simulink model "fourWheelRobotControl_v1"  (R2020b)
settings: Solver=ode3  StartTime=0.0  StopTime=tf  FixedStep=0.0001  RelTol=1e-4  EnableMultiTasking=on
values from neighbouring files (symbols this model uses):
  k_E = 1    [main_robot_control_simulation.m]
  p = [0.127,0.7,0.7,25,0.68,0.001,0.99,0.015,Kt,0.002*Kt,0.56*Kt,     0.00024*Kt,100,0.01,19.2,0,pi/4,-pi/4,pi/4,-pi/4,0,0,0,0]    [main_robot_control_simulation.m]
libraries: pid_lib x7
settings Model: Creator=Sarot PC  LastModifiedBy=ONLY-GOD
settings DataIOCC: LimitDataPoints=on  SaveFormat=Array  ReturnWorkspaceOutputs=off
settings OptimizationCC: LifeSpan=inf
settings DebuggingCC: SolverPrmCheckMsg=warning  InheritedTsInSrcMsg=none  TasksWithSamePriorityMsg=none  SigSpecEnsureSampleTimeMsg=none  ParameterOverflowMsg=none  SignalLabelMismatchMsg=warning  SFUnexpectedBacktrackingDiag=warning  SFNoUnconditionalDefaultTransitionDiag=warning  SFExecutionAtInitializationDiag=none  ArithmeticOperatorsInVariantConditions=warning
settings HardwareCC: ProdBitPerPointer=32  ProdBitPerSizeT=32  ProdBitPerPtrDiffT=32  ProdLargestAtomicFloat=None  ProdIntDivRoundTo=Undefined  ProdEndianess=Unspecified  ProdWordSize=32  ProdHWDeviceType=32-bit Generic
settings ModelReferenceCC: PropagateSignalLabelsOutOfModel=off
settings SFSimCC: SimUseLocalCustomCode=off  CustomCodeUndefinedFunction=UseInterfaceOnly
settings RTWCC: RTWUseLocalCustomCode=off
settings CodeAppCC: StateflowObjectComments=on
settings GRTTargetCC: TargetLangStandard=C89/C90 (ANSI)
settings ConfigComp: CovMetricSettings=dw  CovSaveCumulativeToWorkspaceVar=on  CovSaveSingleToWorkspaceVar=on  CovExternalEMLEnable=off  CovSFcnEnable=off

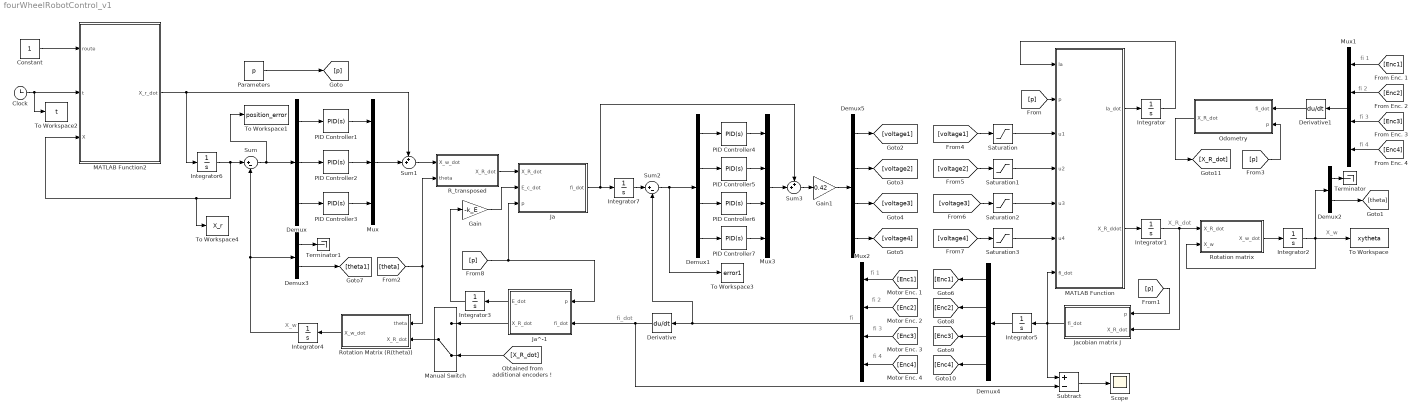
== system fourWheelRobotControl_v1 ==
  note: fi 4
  note: fi 3
  note: fi 2
  note: fi 1
  note: fi_dot
  note: fi
  note: X_w
  note: X_w
  note: X_R_dot
  note: fi 4
  note: fi 3
  note: fi 2
  note: fi 1
  Clock : Clock
  Constant : Constant
  Demux : Demux  Outputs=3
  Demux1 : Demux
  Demux2 : Demux  Outputs=[2,1]
  Demux3 : Demux  Outputs=[2,1]
  Demux4 : Demux
  Demux5 : Demux
  Derivative : Derivative  CoefficientInTFapproximation=0.01
  Derivative1 : Derivative  CoefficientInTFapproximation=0.01
  Gain : Gain  Gain=-k_E
  Gain1 : Gain  Gain=0.42
  Integrator : Integrator  InitialCondition=[0;0;0;0]
  Integrator{1..2,4,6} (4 alike) : Integrator  InitialCondition=[0;0;0]
  Integrator3 : Integrator
  Integrator5 : Integrator  InitialCondition=[0;0;0;0]
  Integrator7 : Integrator  InitialCondition=[0;0;0;0]
  Ja : MATLAB Function  TreatAsAtomicUnit=on
  Ja^-1 : MATLAB Function  TreatAsAtomicUnit=on
  Jacobian matrix J : MATLAB Function  TreatAsAtomicUnit=on
  MATLAB Function : MATLAB Function  TreatAsAtomicUnit=on
  MATLAB Function2 : MATLAB Function  TreatAsAtomicUnit=on
  Manual Switch : ManualSwitch  CurrentSetting=0
  Mux : Mux  Inputs=3
  Mux1 : Mux
  Mux2 : Mux
  Mux3 : Mux
  Odometry : MATLAB Function  TreatAsAtomicUnit=on
  PID Controller1 : pid_lib/PID Controller  Controller=PID  Form=Parallel  TimeDomain=Continuous-time  UseExternalTs=off  SampleTime=-1  IntegratorMethod=Forward Euler  FilterMethod=Forward Euler  ControllerParametersSource=internal  P=5  I=5  D=0  UseFilter=on  N=1000  TunerSelectOption=Transfer Function Based (PID Tuner App)  InitialConditionSource=internal  InitialConditionForIntegrator=0  InitialConditionForFilter=0  DifferentiatorICPrevScaledInput=0  ExternalReset=none  TrackingMode=off  Kt=1  LimitOutput=off  SatLimitsSource=internal  UpperSaturationLimit=inf  LowerSaturationLimit=-inf  LinearizeAsGain=on  AntiWindupMode=none  Kb=1  POutMin=[]  POutMax=[]  IOutMin=[]  IOutMax=[]  DOutMin=[]  DOutMax=[]  NOutMin=[]  NOutMax=[]  SumOutMin=[]  SumOutMax=[]  SaturationOutMin=[]  SaturationOutMax=[]  PParamMin=[]  PParamMax=[]  IParamMin=[]  IParamMax=[]  DParamMin=[]  DParamMax=[]  NParamMin=[]  NParamMax=[]  KbParamMin=[]  KbParamMax=[]  KtParamMin=[]  KtParamMax=[]  KbOutMin=[]  KbOutMax=[]  KtOutMin=[]  KtOutMax=[]  IntegratorOutMin=[]  IntegratorOutMax=[]  FilterOutMin=[]  FilterOutMax=[]  SumI1OutMin=[]  SumI1OutMax=[]  SumI2OutMin=[]  SumI2OutMax=[]  SumI3OutMin=[]  SumI3OutMax=[]  SumI4OutMin=[]  SumI4OutMax=[]  SumDOutMin=[]  SumDOutMax=[]  DifferentiatorOutMin=[]  DifferentiatorOutMax=[]  FilterDiffOutCoefMin=[]  FilterDiffOutCoefMax=[]  ReciprocalOutMin=[]  ReciprocalOutMax=[]  SumDenOutMin=[]  SumDenOutMax=[]  SumNumOutMin=[]  SumNumOutMax=[]  DivideOutMin=[]  DivideOutMax=[]  UdiffTsProdOutMin=[]  UdiffTsProdOutMax=[]  NTsProdOutMin=[]  NTsProdOutMax=[]  UintegralTsProdOutMin=[]  UintegralTsProdOutMax=[]  UngainTsProdOutMin=[]  UngainTsProdOutMax=[]  IntegratorContinuousStateAttributes=''  IntegratorStateMustResolveToSignalObject=off  IntegratorRTWStateStorageClass=Auto  FilterContinuousStateAttributes=''  FilterStateMustResolveToSignalObject=off  FilterRTWStateStorageClass=Auto  ParallelPVariant=InternalParameters  IdealPVariant=Disabled  IVariant=InternalParameters  DVariant=InternalParameters  IntegratorVariant=Continuous  SatVariant=Disabled  AWVariant=Passthrough  PCopyVariant=Disabled  TRVariant=Disabled  FdbkBlocksVariant=Forward  IdealPFdbkVariant=Disabled  SatFdbkVariant=Disabled  DerivativeFilterVariant=ContFilter  NVariant=InternalParameters  NCopyVariant=Disabled  FilterICVariant=InternalICsFilter  IntegratorICVariant=InternalICs  ExternalResetVariant=Disabled  TRSumVariant=Passthrough  SumFdbkVariant=Disabled  SumVariant=Sum_PID  TsampFilterVariant=InternalTs  TsampNgainVariant=Passthrough  TsampIntegralVariant=Passthrough  ExternalSaturationOutDataTypeStr=Inherit: Same as second input
  PID Controller2 : pid_lib/PID Controller  Controller=PID  Form=Parallel  TimeDomain=Continuous-time  UseExternalTs=off  SampleTime=-1  IntegratorMethod=Forward Euler  FilterMethod=Forward Euler  ControllerParametersSource=internal  P=5  I=5  D=0  UseFilter=on  N=1000  TunerSelectOption=Transfer Function Based (PID Tuner App)  InitialConditionSource=internal  InitialConditionForIntegrator=0  InitialConditionForFilter=0  DifferentiatorICPrevScaledInput=0  ExternalReset=none  TrackingMode=off  Kt=1  LimitOutput=off  SatLimitsSource=internal  UpperSaturationLimit=inf  LowerSaturationLimit=-inf  LinearizeAsGain=on  AntiWindupMode=none  Kb=1  POutMin=[]  POutMax=[]  IOutMin=[]  IOutMax=[]  DOutMin=[]  DOutMax=[]  NOutMin=[]  NOutMax=[]  SumOutMin=[]  SumOutMax=[]  SaturationOutMin=[]  SaturationOutMax=[]  PParamMin=[]  PParamMax=[]  IParamMin=[]  IParamMax=[]  DParamMin=[]  DParamMax=[]  NParamMin=[]  NParamMax=[]  KbParamMin=[]  KbParamMax=[]  KtParamMin=[]  KtParamMax=[]  KbOutMin=[]  KbOutMax=[]  KtOutMin=[]  KtOutMax=[]  IntegratorOutMin=[]  IntegratorOutMax=[]  FilterOutMin=[]  FilterOutMax=[]  SumI1OutMin=[]  SumI1OutMax=[]  SumI2OutMin=[]  SumI2OutMax=[]  SumI3OutMin=[]  SumI3OutMax=[]  SumI4OutMin=[]  SumI4OutMax=[]  SumDOutMin=[]  SumDOutMax=[]  DifferentiatorOutMin=[]  DifferentiatorOutMax=[]  FilterDiffOutCoefMin=[]  FilterDiffOutCoefMax=[]  ReciprocalOutMin=[]  ReciprocalOutMax=[]  SumDenOutMin=[]  SumDenOutMax=[]  SumNumOutMin=[]  SumNumOutMax=[]  DivideOutMin=[]  DivideOutMax=[]  UdiffTsProdOutMin=[]  UdiffTsProdOutMax=[]  NTsProdOutMin=[]  NTsProdOutMax=[]  UintegralTsProdOutMin=[]  UintegralTsProdOutMax=[]  UngainTsProdOutMin=[]  UngainTsProdOutMax=[]  IntegratorContinuousStateAttributes=''  IntegratorStateMustResolveToSignalObject=off  IntegratorRTWStateStorageClass=Auto  FilterContinuousStateAttributes=''  FilterStateMustResolveToSignalObject=off  FilterRTWStateStorageClass=Auto  ParallelPVariant=InternalParameters  IdealPVariant=Disabled  IVariant=InternalParameters  DVariant=InternalParameters  IntegratorVariant=Continuous  SatVariant=Disabled  AWVariant=Passthrough  PCopyVariant=Disabled  TRVariant=Disabled  FdbkBlocksVariant=Forward  IdealPFdbkVariant=Disabled  SatFdbkVariant=Disabled  DerivativeFilterVariant=ContFilter  NVariant=InternalParameters  NCopyVariant=Disabled  FilterICVariant=InternalICsFilter  IntegratorICVariant=InternalICs  ExternalResetVariant=Disabled  TRSumVariant=Passthrough  SumFdbkVariant=Disabled  SumVariant=Sum_PID  TsampFilterVariant=InternalTs  TsampNgainVariant=Passthrough  TsampIntegralVariant=Passthrough  ExternalSaturationOutDataTypeStr=Inherit: Same as second input
  PID Controller3 : pid_lib/PID Controller  Controller=PID  Form=Parallel  TimeDomain=Continuous-time  UseExternalTs=off  SampleTime=-1  IntegratorMethod=Forward Euler  FilterMethod=Forward Euler  ControllerParametersSource=internal  P=5  I=5  D=0  UseFilter=on  N=1000  TunerSelectOption=Transfer Function Based (PID Tuner App)  InitialConditionSource=internal  InitialConditionForIntegrator=0  InitialConditionForFilter=0  DifferentiatorICPrevScaledInput=0  ExternalReset=none  TrackingMode=off  Kt=1  LimitOutput=off  SatLimitsSource=internal  UpperSaturationLimit=inf  LowerSaturationLimit=-inf  LinearizeAsGain=on  AntiWindupMode=none  Kb=1  POutMin=[]  POutMax=[]  IOutMin=[]  IOutMax=[]  DOutMin=[]  DOutMax=[]  NOutMin=[]  NOutMax=[]  SumOutMin=[]  SumOutMax=[]  SaturationOutMin=[]  SaturationOutMax=[]  PParamMin=[]  PParamMax=[]  IParamMin=[]  IParamMax=[]  DParamMin=[]  DParamMax=[]  NParamMin=[]  NParamMax=[]  KbParamMin=[]  KbParamMax=[]  KtParamMin=[]  KtParamMax=[]  KbOutMin=[]  KbOutMax=[]  KtOutMin=[]  KtOutMax=[]  IntegratorOutMin=[]  IntegratorOutMax=[]  FilterOutMin=[]  FilterOutMax=[]  SumI1OutMin=[]  SumI1OutMax=[]  SumI2OutMin=[]  SumI2OutMax=[]  SumI3OutMin=[]  SumI3OutMax=[]  SumI4OutMin=[]  SumI4OutMax=[]  SumDOutMin=[]  SumDOutMax=[]  DifferentiatorOutMin=[]  DifferentiatorOutMax=[]  FilterDiffOutCoefMin=[]  FilterDiffOutCoefMax=[]  ReciprocalOutMin=[]  ReciprocalOutMax=[]  SumDenOutMin=[]  SumDenOutMax=[]  SumNumOutMin=[]  SumNumOutMax=[]  DivideOutMin=[]  DivideOutMax=[]  UdiffTsProdOutMin=[]  UdiffTsProdOutMax=[]  NTsProdOutMin=[]  NTsProdOutMax=[]  UintegralTsProdOutMin=[]  UintegralTsProdOutMax=[]  UngainTsProdOutMin=[]  UngainTsProdOutMax=[]  IntegratorContinuousStateAttributes=''  IntegratorStateMustResolveToSignalObject=off  IntegratorRTWStateStorageClass=Auto  FilterContinuousStateAttributes=''  FilterStateMustResolveToSignalObject=off  FilterRTWStateStorageClass=Auto  ParallelPVariant=InternalParameters  IdealPVariant=Disabled  IVariant=InternalParameters  DVariant=InternalParameters  IntegratorVariant=Continuous  SatVariant=Disabled  AWVariant=Passthrough  PCopyVariant=Disabled  TRVariant=Disabled  FdbkBlocksVariant=Forward  IdealPFdbkVariant=Disabled  SatFdbkVariant=Disabled  DerivativeFilterVariant=ContFilter  NVariant=InternalParameters  NCopyVariant=Disabled  FilterICVariant=InternalICsFilter  IntegratorICVariant=InternalICs  ExternalResetVariant=Disabled  TRSumVariant=Passthrough  SumFdbkVariant=Disabled  SumVariant=Sum_PID  TsampFilterVariant=InternalTs  TsampNgainVariant=Passthrough  TsampIntegralVariant=Passthrough  ExternalSaturationOutDataTypeStr=Inherit: Same as second input
  PID Controller{4..7} (4 alike) : pid_lib/PID Controller  Controller=PID  Form=Parallel  TimeDomain=Continuous-time  UseExternalTs=off  SampleTime=-1  IntegratorMethod=Forward Euler  FilterMethod=Forward Euler  ControllerParametersSource=internal  P=100  I=0  D=30  UseFilter=on  N=1000  TunerSelectOption=Transfer Function Based (PID Tuner App)  InitialConditionSource=internal  InitialConditionForIntegrator=0  InitialConditionForFilter=0  DifferentiatorICPrevScaledInput=0  ExternalReset=none  TrackingMode=off  Kt=1  LimitOutput=off  SatLimitsSource=internal  UpperSaturationLimit=inf  LowerSaturationLimit=-inf  LinearizeAsGain=on  AntiWindupMode=none  Kb=1  POutMin=[]  POutMax=[]  IOutMin=[]  IOutMax=[]  DOutMin=[]  DOutMax=[]  NOutMin=[]  NOutMax=[]  SumOutMin=[]  SumOutMax=[]  SaturationOutMin=[]  SaturationOutMax=[]  PParamMin=[]  PParamMax=[]  IParamMin=[]  IParamMax=[]  DParamMin=[]  DParamMax=[]  NParamMin=[]  NParamMax=[]  KbParamMin=[]  KbParamMax=[]  KtParamMin=[]  KtParamMax=[]  KbOutMin=[]  KbOutMax=[]  KtOutMin=[]  KtOutMax=[]  IntegratorOutMin=[]  IntegratorOutMax=[]  FilterOutMin=[]  FilterOutMax=[]  SumI1OutMin=[]  SumI1OutMax=[]  SumI2OutMin=[]  SumI2OutMax=[]  SumI3OutMin=[]  SumI3OutMax=[]  SumI4OutMin=[]  SumI4OutMax=[]  SumDOutMin=[]  SumDOutMax=[]  DifferentiatorOutMin=[]  DifferentiatorOutMax=[]  FilterDiffOutCoefMin=[]  FilterDiffOutCoefMax=[]  ReciprocalOutMin=[]  ReciprocalOutMax=[]  SumDenOutMin=[]  SumDenOutMax=[]  SumNumOutMin=[]  SumNumOutMax=[]  DivideOutMin=[]  DivideOutMax=[]  UdiffTsProdOutMin=[]  UdiffTsProdOutMax=[]  NTsProdOutMin=[]  NTsProdOutMax=[]  UintegralTsProdOutMin=[]  UintegralTsProdOutMax=[]  UngainTsProdOutMin=[]  UngainTsProdOutMax=[]  IntegratorContinuousStateAttributes=''  IntegratorStateMustResolveToSignalObject=off  IntegratorRTWStateStorageClass=Auto  FilterContinuousStateAttributes=''  FilterStateMustResolveToSignalObject=off  FilterRTWStateStorageClass=Auto  ParallelPVariant=InternalParameters  IdealPVariant=Disabled  IVariant=InternalParameters  DVariant=InternalParameters  IntegratorVariant=Continuous  SatVariant=Disabled  AWVariant=Passthrough  PCopyVariant=Disabled  TRVariant=Disabled  FdbkBlocksVariant=Forward  IdealPFdbkVariant=Disabled  SatFdbkVariant=Disabled  DerivativeFilterVariant=ContFilter  NVariant=InternalParameters  NCopyVariant=Disabled  FilterICVariant=InternalICsFilter  IntegratorICVariant=InternalICs  ExternalResetVariant=Disabled  TRSumVariant=Passthrough  SumFdbkVariant=Disabled  SumVariant=Sum_PID  TsampFilterVariant=InternalTs  TsampNgainVariant=Passthrough  TsampIntegralVariant=Passthrough  ExternalSaturationOutDataTypeStr=Inherit: Same as second input
  Parameters : Constant  Value=p
  R_transposed : MATLAB Function  TreatAsAtomicUnit=on
  Rotation Matrix (R(theta)) : MATLAB Function  TreatAsAtomicUnit=on
  Rotation matrix : MATLAB Function  TreatAsAtomicUnit=on
  Saturation{,1..3} (4 alike) : Saturate  UpperLimit=24  LowerLimit=-24
  Scope : Scope
  Subtract : Sum  Inputs=+-
  Sum : Sum  Inputs=|+-
  Sum1 : Sum  Inputs=++|
  Sum2 : Sum  Inputs=|+-
  Sum3 : Sum  Inputs=++|
  Terminator : Terminator
  Terminator1 : Terminator
  To Workspace : ToWorkspace  VariableName=xytheta  SampleTime=-1
  To Workspace1 : ToWorkspace  VariableName=position_error  SampleTime=-1
  To Workspace2 : ToWorkspace  VariableName=t  SampleTime=-1
  To Workspace3 : ToWorkspace  VariableName=error1  SampleTime=-1
  To Workspace4 : ToWorkspace  VariableName=X_r  SampleTime=-1
  wires:
  [p] -> MATLAB Function/2(p)
  MATLAB Function/1(Ia_dot) -> Integrator/1
  MATLAB Function/2(X_R_ddot) -> Integrator1/1
  Integrator1/1 -> Jacobian matrix J/2(X_R_dot), Rotation matrix/1(X_R_dot)
  Rotation matrix/1(X_w_dot) -> Integrator2/1
  Jacobian matrix J/1(fi_dot) -> Subtract/1, Integrator5/1, MATLAB Function/7(fi_dot)
  Integrator/1 -> MATLAB Function/1(Ia)
  Integrator2/1 -> Rotation matrix/2(X_w), Demux2/1, To Workspace/1
  Parameters/1 -> [p]
  [p] -> Jacobian matrix J/1(p)
  Saturation/1 -> MATLAB Function/3(u1)
  [voltage1] -> Saturation/1
  Saturation1/1 -> MATLAB Function/4(u2)
  [voltage2] -> Saturation1/1
  Saturation2/1 -> MATLAB Function/5(u3)
  [voltage3] -> Saturation2/1
  Saturation3/1 -> MATLAB Function/6(u4)
  [voltage4] -> Saturation3/1
  Sum/1 -> To Workspace1/1, Demux/1
  Mux/1 -> Sum1/2
  Sum1/1 -> R_transposed/1(X_w_dot)
  R_transposed/1(X_R_dot) -> Ja/1(X_R_dot)
  Ja/1(fi_dot) -> Sum3/1, Integrator7/1
  PID Controller1/1 -> Mux/1
  PID Controller2/1 -> Mux/2
  PID Controller3/1 -> Mux/3
  Demux/1 -> PID Controller1/1
  Demux/2 -> PID Controller2/1
  Demux/3 -> PID Controller3/1
  Sum2/1 -> Demux1/1, To Workspace3/1
  Demux1/1 -> PID Controller4/1
  Demux1/2 -> PID Controller5/1
  Demux1/3 -> PID Controller6/1
  Demux1/4 -> PID Controller7/1
  MATLAB Function2/1(X_r_dot) -> Integrator6/1, Sum1/1
  [theta] -> Rotation Matrix (R(theta))/1(theta), R_transposed/2(theta)
  Gain/1 -> Ja/2(E_c_dot)
  Ja^-1/1(E_dot) -> Integrator3/1
  Integrator3/1 -> Gain/1
  Rotation Matrix (R(theta))/1(X_w_dot) -> Integrator4/1
  Integrator4/1 -> Sum/2, Demux3/1
  Derivative/1 -> Ja^-1/2(fi_dot), Subtract/2
  Demux2/2 -> [theta]
  Demux2/1 -> Terminator/1
  [p] -> Ja/3(p), Ja^-1/1(p)
  [Enc1] -> Mux1/1
  [Enc2] -> Mux1/2
  [Enc3] -> Mux1/3
  [Enc4] -> Mux1/4
  Mux1/1 -> Derivative1/1
  Odometry/1(X_R_dot) -> [X_R_dot]
  Derivative1/1 -> Odometry/1(fi_dot)
  [Enc1] -> Mux2/1
  [Enc2] -> Mux2/2
  [Enc3] -> Mux2/3
  [Enc4] -> Mux2/4
  Mux2/1 -> Sum2/2, Derivative/1
  Integrator5/1 -> Demux4/1
  Demux4/1 -> [Enc1]
  Demux4/2 -> [Enc2]
  Demux4/3 -> [Enc3]
  Demux4/4 -> [Enc4]
  [p] -> Odometry/2(p)
  Demux3/1 -> Terminator1/1
  Demux3/2 -> [theta1]
  Ja^-1/2(X_R_dot) -> Manual Switch/1
  Manual Switch/1 -> Rotation Matrix (R(theta))/2(X_R_dot)
  [X_R_dot] -> Manual Switch/2
  Clock/1 -> MATLAB Function2/2(t), To Workspace2/1
  Constant/1 -> MATLAB Function2/1(route)
  Integrator6/1 -> To Workspace4/1, MATLAB Function2/3(X), Sum/1
  Subtract/1 -> Scope/1
  Integrator7/1 -> Sum2/1
  PID Controller4/1 -> Mux3/1
  PID Controller5/1 -> Mux3/2
  PID Controller6/1 -> Mux3/3
  PID Controller7/1 -> Mux3/4
  Mux3/1 -> Sum3/2
  Sum3/1 -> Gain1/1
  Gain1/1 -> Demux5/1
  Demux5/1 -> [voltage1]
  Demux5/2 -> [voltage2]
  Demux5/3 -> [voltage3]
  Demux5/4 -> [voltage4]

== matlab function fourWheelRobotControl_v1/Jacobian matrix J ==
  data: p input; X_R_dot input; fi_dot output
function fi_dot = fcn(p,X_R_dot)
%#codegen
w_d = p(1);         % wheel diameter
r = w_d/2;          % wheel radius
robot_w = p(2);     % robot width
robot_l = p(3);     % robot length
a = robot_w/2;
b = robot_l/2;
l = sqrt(a^2+b^2);
% m = p(4);           % robot mass
% I_robot = p(5);     % robot inertia
% La = p(6);          % motor inductance
% Ra = p(7);          % motor resistor
% Kb = p(8);          % motor back emf
% Kt = p(9);          % Torque constant
% J1 = p(10)*Kt;      % motor rotor inertia
% Tc = p(11)*Kt;      % Coulomb friction
% D = p(12)*Kt;       % viscous coefficient
% k = p(13);          % appr. friction slope
% eps = p(14);        % angular rate threshold
% n_G = p(15);        % gear ratio
% J2 = p(16)*Kt;      % gear inertia
alpha_1 = -atan(a/b);    %
alpha_2 = atan(a/b);    %
alpha_3 = pi/2+atan(a/b);    %
alpha_4 = -pi/2-atan(a/b);    %
delta_1 = p(17);    %
delta_2 = p(18);    %
delta_3 = p(19);    %
delta_4 = p(20);    %
gamma_1 = p(21);    %
gamma_2 = p(22);    %
gamma_3 = p(23);    %
gamma_4 = p(24);    %
J = zeros(4,3);
J(1,:) = (r*cos(gamma_1))\[cos(delta_1+gamma_1),...
        sin(delta_1+gamma_1), l*sin(delta_1+gamma_1-alpha_1)];
J(2,:) = (r*cos(gamma_2))\[cos(delta_2+gamma_2),...
        sin(delta_2+gamma_2), l*sin(delta_2+gamma_2-alpha_2)];
J(3,:) = (r*cos(gamma_3))\[cos(delta_3+gamma_3),...
        sin(delta_3+gamma_3), l*sin(delta_3+gamma_3-alpha_3)];
J(4,:) = (r*cos(gamma_4))\[cos(delta_4+gamma_4),...
        sin(delta_4+gamma_4), l*sin(delta_4+gamma_4-alpha_4)];

fi_dot = J*X_R_dot;

== matlab function fourWheelRobotControl_v1/MATLAB Function ==
  data: Ia input; p input; Ia_dot output; u1 input; u2 input; u3 input; u4 input; X_R_ddot output; fi_dot input
function [Ia_dot,X_R_ddot] = fcn(Ia,p,u1,u2,u3,u4,fi_dot)
%#codegen
w_d = p(1);         % wheel diameter
r = w_d/2;          % wheel radius
robot_w = p(2);     % robot width
robot_l = p(3);     % robot length
a = robot_w/2;
b = robot_l/2;
l = sqrt(a^2+b^2);
m = p(4);           % robot mass
I_robot = p(5);     % robot inertia
La = p(6);          % motor inductance
Ra = p(7);          % motor resistor
Kb = p(8);          % motor back emf
Kt = p(9);          % Torque constant
J1 = p(10)*Kt;      % motor rotor inertia
Tc = p(11)*Kt;      % Coulomb friction
D = p(12)*Kt;       % viscous coefficient
% k = p(13);          % appr. friction slope
eps = p(14);        % angular rate threshold
n_G = p(15);        % gear ratio
J2 = p(16)*Kt;      % gear inertia
alpha_1 = -atan(a/b);    %
alpha_2 = atan(a/b);    %
alpha_3 = pi/2+atan(a/b);    %
alpha_4 = -pi/2-atan(a/b);    %
delta_1 = p(17);    %
delta_2 = p(18);    %
delta_3 = p(19);    %
delta_4 = p(20);    %
gamma_1 = p(21);    %
gamma_2 = p(22);    %
gamma_3 = p(23);    %
gamma_4 = p(24);    %

I_i = J2*1/n_G+J1*n_G; % total motor inertia

u = [u1;u2;u3;u4];
Ia_dot = La\(-Ra*Ia-Kb*n_G*fi_dot+u);

H = diag([m,m,I_robot]);
J = zeros(4,3);
J(1,:) = (r*cos(gamma_1))\[cos(delta_1+gamma_1),...
        sin(delta_1+gamma_1), l*sin(delta_1+gamma_1-alpha_1)];
J(2,:) = (r*cos(gamma_2))\[cos(delta_2+gamma_2),...
        sin(delta_2+gamma_2), l*sin(delta_2+gamma_2-alpha_2)];
J(3,:) = (r*cos(gamma_3))\[cos(delta_3+gamma_3),...
        sin(delta_3+gamma_3), l*sin(delta_3+gamma_3-alpha_3)];
J(4,:) = (r*cos(gamma_4))\[cos(delta_4+gamma_4),...
        sin(delta_4+gamma_4), l*sin(delta_4+gamma_4-alpha_4)];

Mfric = zeros(4,1);
for i=1:4
    if abs(fi_dot(i))<eps
        Mfric(i) = (Tc+D*eps)/eps*fi_dot(i);
    else
        Mfric(i) = Tc*sign(fi_dot(i))+D*fi_dot(i);
    end
end

X_R_ddot = (H/n_G+I_i*(J'*J))\(-J'*Mfric+Kt*J'*Ia);
end

== matlab function fourWheelRobotControl_v1/Rotation matrix ==
  data: X_R_dot input; X_w_dot output; X_w input
function X_w_dot = fcn(X_R_dot,X_w)
%#codegen
theta = X_w(3);
R = [cos(theta) -sin(theta) 0;
     sin(theta)  cos(theta) 0;
         0          0       1];
X_w_dot = R*X_R_dot;

== matlab function fourWheelRobotControl_v1/R_transposed ==
  data: X_w_dot input; X_R_dot output; theta input
function X_R_dot = fcn(X_w_dot,theta)
%#codegen

R__T = [cos(theta) sin(theta) 0;-sin(theta) cos(theta) 0;0 0 1];
X_R_dot = R__T*X_w_dot;

== matlab function fourWheelRobotControl_v1/Ja ==
  data: X_R_dot input; E_c_dot input; p input; fi_dot output
function fi_dot = fcn(X_R_dot,E_c_dot,p)
%#codegen

w_d = p(1);         % wheel diameter
r = w_d/2;          % wheel radius
robot_w = p(2);     % robot width
robot_l = p(3);     % robot length
a = robot_w/2;
b = robot_l/2;
l = sqrt(a^2+b^2);
% m = p(4);           % robot mass
% I_robot = p(5);     % robot inertia
% La = p(6);          % motor inductance
% Ra = p(7);          % motor resistor
% Kb = p(8);          % motor back emf
% Kt = p(9);          % Torque constant
% J1 = p(10)*Kt;      % motor rotor inertia
% Tc = p(11)*Kt;      % Coulomb friction
% D = p(12)*Kt;       % viscous coefficient
% k = p(13);          % appr. friction slope
% eps = p(14);        % angular rate threshold
% n_G = p(15);        % gear ratio
% J2 = p(16)*Kt;      % gear inertia
alpha_1 = -atan(a/b);    %
alpha_2 = atan(a/b);    %
alpha_3 = pi/2+atan(a/b);    %
alpha_4 = -pi/2-atan(a/b);    %
delta_1 = p(17);    %
delta_2 = p(18);    %
delta_3 = p(19);    %
delta_4 = p(20);    %
gamma_1 = p(21);    %
gamma_2 = p(22);    %
gamma_3 = p(23);    %
gamma_4 = p(24);    %
J = zeros(4,3);
J(1,:) = (r*cos(gamma_1))\[cos(delta_1+gamma_1),...
        sin(delta_1+gamma_1), l*sin(delta_1+gamma_1-alpha_1)];
J(2,:) = (r*cos(gamma_2))\[cos(delta_2+gamma_2),...
        sin(delta_2+gamma_2), l*sin(delta_2+gamma_2-alpha_2)];
J(3,:) = (r*cos(gamma_3))\[cos(delta_3+gamma_3),...
        sin(delta_3+gamma_3), l*sin(delta_3+gamma_3-alpha_3)];
J(4,:) = (r*cos(gamma_4))\[cos(delta_4+gamma_4),...
        sin(delta_4+gamma_4), l*sin(delta_4+gamma_4-alpha_4)];
J_dager = (J'*J)\J';
J3 = J(1:3,:); Jm = J(4:end,:); [m,~]=size(Jm);
T = [Jm/J3 -eye(m)];
Ja_inv = [J_dager;T];
X_a_dot = [X_R_dot;E_c_dot];
fi_dot = Ja_inv\X_a_dot;

== matlab function fourWheelRobotControl_v1/Rotation Matrix (R(theta)) ==
  data: theta input; X_w_dot output; X_R_dot input
function X_w_dot = fcn(theta,X_R_dot)
%#codegen

R = [cos(theta) -sin(theta) 0; sin(theta) cos(theta) 0; 0 0 1];
X_w_dot = R*X_R_dot;

== matlab function fourWheelRobotControl_v1/Ja^-1 ==
  data: p input; E_dot output; X_R_dot output; fi_dot input
function [E_dot,X_R_dot] = fcn(p,fi_dot)
%#codegen

w_d = p(1);         % wheel diameter
r = w_d/2;          % wheel radius
robot_w = p(2);     % robot width
robot_l = p(3);     % robot length
a = robot_w/2;
b = robot_l/2;
l = sqrt(a^2+b^2);
% m = p(4);           % robot mass
% I_robot = p(5);     % robot inertia
% La = p(6);          % motor inductance
% Ra = p(7);          % motor resistor
% Kb = p(8);          % motor back emf
% Kt = p(9);          % Torque constant
% J1 = p(10)*Kt;      % motor rotor inertia
% Tc = p(11)*Kt;      % Coulomb friction
% D = p(12)*Kt;       % viscous coefficient
% k = p(13);          % appr. friction slope
% eps = p(14);        % angular rate threshold
% n_G = p(15);        % gear ratio
% J2 = p(16)*Kt;      % gear inertia
alpha_1 = -atan(a/b);    %
alpha_2 = atan(a/b);    %
alpha_3 = pi/2+atan(a/b);    %
alpha_4 = -pi/2-atan(a/b);    %
delta_1 = p(17);    %
delta_2 = p(18);    %
delta_3 = p(19);    %
delta_4 = p(20);    %
gamma_1 = p(21);    %
gamma_2 = p(22);    %
gamma_3 = p(23);    %
gamma_4 = p(24);    %
J = zeros(4,3);
J(1,:) = (r*cos(gamma_1))\[cos(delta_1+gamma_1),...
        sin(delta_1+gamma_1), l*sin(delta_1+gamma_1-alpha_1)];
J(2,:) = (r*cos(gamma_2))\[cos(delta_2+gamma_2),...
        sin(delta_2+gamma_2), l*sin(delta_2+gamma_2-alpha_2)];
J(3,:) = (r*cos(gamma_3))\[cos(delta_3+gamma_3),...
        sin(delta_3+gamma_3), l*sin(delta_3+gamma_3-alpha_3)];
J(4,:) = (r*cos(gamma_4))\[cos(delta_4+gamma_4),...
        sin(delta_4+gamma_4), l*sin(delta_4+gamma_4-alpha_4)];
J_dager = (J'*J)\J';
J3 = J(1:3,:); Jm = J(4:end,:); [m,~]=size(Jm);
T = [Jm/J3 -eye(m)];
Ja_inv = [J_dager;T];
X_a_dot = Ja_inv*fi_dot;
X_R_dot = X_a_dot(1:3);
E_dot = X_a_dot(4:end);

== matlab function fourWheelRobotControl_v1/Odometry ==
  data: fi_dot input; X_R_dot output; p input
function X_R_dot = fcn(fi_dot,p)
%#codegen

w_d = p(1);         % wheel diameter
r = w_d/2;          % wheel radius
robot_w = p(2);     % robot width
robot_l = p(3);     % robot length
a = robot_w/2;
b = robot_l/2;
l = sqrt(a^2+b^2);
% m = p(4);           % robot mass
% I_robot = p(5);     % robot inertia
% La = p(6);          % motor inductance
% Ra = p(7);          % motor resistor
% Kb = p(8);          % motor back emf
% Kt = p(9);          % Torque constant
% J1 = p(10)*Kt;      % motor rotor inertia
% Tc = p(11)*Kt;      % Coulomb friction
% D = p(12)*Kt;       % viscous coefficient
% k = p(13);          % appr. friction slope
% eps = p(14);        % angular rate threshold
% n_G = p(15);        % gear ratio
% J2 = p(16)*Kt;      % gear inertia
alpha_1 = -atan(a/b);    %
alpha_2 = atan(a/b);    %
alpha_3 = pi/2+atan(a/b);    %
alpha_4 = -pi/2-atan(a/b);    %
delta_1 = p(17);    %
delta_2 = p(18);    %
delta_3 = p(19);    %
delta_4 = p(20);    %
gamma_1 = p(21);    %
gamma_2 = p(22);    %
gamma_3 = p(23);    %
gamma_4 = p(24);    %
J = zeros(4,3);
J(1,:) = (r*cos(gamma_1))\[cos(delta_1+gamma_1),...
        sin(delta_1+gamma_1), l*sin(delta_1+gamma_1-alpha_1)];
J(2,:) = (r*cos(gamma_2))\[cos(delta_2+gamma_2),...
        sin(delta_2+gamma_2), l*sin(delta_2+gamma_2-alpha_2)];
J(3,:) = (r*cos(gamma_3))\[cos(delta_3+gamma_3),...
        sin(delta_3+gamma_3), l*sin(delta_3+gamma_3-alpha_3)];
J(4,:) = (r*cos(gamma_4))\[cos(delta_4+gamma_4),...
        sin(delta_4+gamma_4), l*sin(delta_4+gamma_4-alpha_4)];
J_dager = (J'*J)\J';
X_R_dot = J_dager*fi_dot;

== matlab function fourWheelRobotControl_v1/MATLAB Function2 ==
  settings: updateMethod=DISCRETE
  data: route input; t input; X_r_dot output; X input
function X_r_dot = fcn(route,t,X)
%#codegen

persistent k i j X_p_i omega_p_j t1 t2
if isempty(k)
    i = int8(1);
    j = int8(1);
    X_p_i = [0;0];
    omega_p_j = 0;
    t1 = t;
    t2 = t;
    k = 1;
end
tau = 0.15;
tau1 = 0.15;
V_max = 2; % maximum velocity
a = 1;      % acceleration
omega_max = 1.5;
alpha = 1;

X_r_dot = zeros(3,1);
switch route
    case 1
%         X_p = [1.5   1.5  0];
        X_p = [1.5   1.5  pi/2
               1.5    3   0
               2     4    0]; % X_p = [x,y,theta];
    otherwise
        X_r_dot = [0;0;0];
        return;
end
X_p = X_p'; % X_p = [x;y;theta]
[~,col] = size(X_p);
dX = X_p(1:2,i)-X_p_i;
norm_dX = norm(dX);
two_rmin = V_max^2/a;
dtheta = X_p(3,j)-omega_p_j;
norm_dtheta = abs(dtheta);
two_thetamin = omega_max^2/alpha;

if norm_dX > two_rmin
    ta = V_max/a;                   % acceleration period
    tad = (norm_dX-two_rmin)/V_max; % acc to deceleration period
    td = ta + tad;                  % start deceleration
    te = ta + td;                   % end deceleration
    if (t-t1) < ta
        v = a*(t-t1);
    elseif ta <= (t-t1) && (t-t1) < td
        v = V_max;
    elseif td <= (t-t1) && (t-t1) < te
        v = -a*(t-t1-td) + V_max;
    else
        v = 0;
    end
else
    tp = sqrt(norm_dX/a);
    te = 2*tp;
    Vp = a*tp;
    if (t-t1) < tp
        v = a*(t-t1);
    elseif tp < (t-t1) && (t-t1) < te
        v = -a*(t-t1-tp)+Vp;
    else
        v = 0;
    end
end
if norm_dX~=0
    X_r_dot(1:2) = v*dX/norm_dX;
end

dist_X = norm(X_p(1:2,i)-X(1:2));
if (i<col)&&(dist_X < tau)
    X_p_i = X(1:2);
    t1    = t;
    i     = i+1;
end

if norm_dtheta > two_thetamin
    ta = omega_max/alpha;                   % acceleration period
    tad = (norm_dtheta-two_thetamin)/omega_max; % acc to deceleration period
    td = ta + tad;                  % start deceleration
    te = ta + td;                   % end deceleration
    if (t-t2) < ta
        omega = alpha*(t-t2);
    elseif ta <= (t-t2) && (t-t2) < td
        omega = omega_max;
    elseif td <= (t-t2) && (t-t2) < te
        omega = -alpha*(t-t2-td) + omega_max;
    else
        omega = 0;
    end
else
    tp = sqrt(norm_dtheta/alpha);
    te = 2*tp;
    omegap = alpha*tp;
    if (t-t2) < tp
        omega = alpha*(t-t2);
    elseif tp < (t-t2) && (t-t2) < te
        omega = -alpha*(t-t2-tp)+omegap;
    else
        omega = 0;
    end
end
X_r_dot(3) = omega*sign(dtheta);

dist_theta = abs(X_p(3,j)-X(3));
if (j<col)&&(dist_theta < tau1)
    omega_p_j = X(3);
    t2    = t;
    j     = j+1;
end
